simulink model "two_dof_arm_with_lqr"  (R2023a)
settings: Solver=FixedStepAuto  StartTime=0.0  StopTime=5  FixedStep=0.001  RelTol=1e-3
InitFcn:
  | two_link_planar_manipulator_sim
values from neighbouring files (symbols this model uses):
  g = [0 -9.81 0]    [two_link_planar_manipulator_sim.m]
  K = lqr(A,B,Q,R)    [two_link_planar_manipulator_sim.m]
  l = [0.25 0.25]    [two_link_planar_manipulator_sim.m]
  m = [1 1]    [two_link_planar_manipulator_sim.m]
  offset_error = 0.0175    [two_link_planar_manipulator_sim.m]
  resolution = 2^12    (= 4096)    [two_link_planar_manipulator_sim.m]
  sample_time = 0.001    [two_link_planar_manipulator_sim.m]
  true_delay = floor(delay*10^-3/sample_time)+sample_time*10^3    [two_link_planar_manipulator_sim.m]
  w = [0.04 0.04]    [two_link_planar_manipulator_sim.m]
  without_actuator_dynamics = true    [two_link_planar_manipulator_sim.m]
  without_meas_uncertainty = false    [two_link_planar_manipulator_sim.m]
libraries: spsFirstOrderFilterLib x2, robotmaniplib x1, simulink x1
settings Model: Creator=Jordan  LastModifiedBy=Jordan

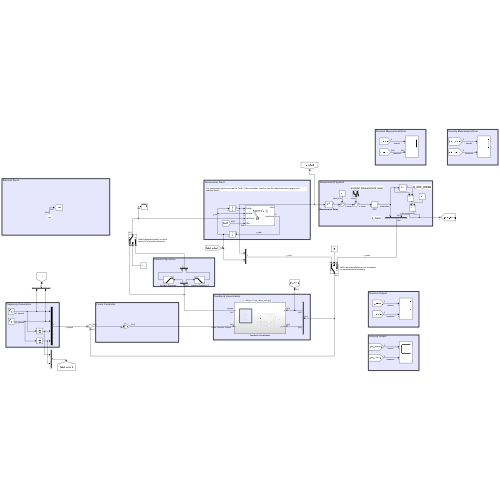
[thumbnail: Simulink's stored preview of the top-level diagram]
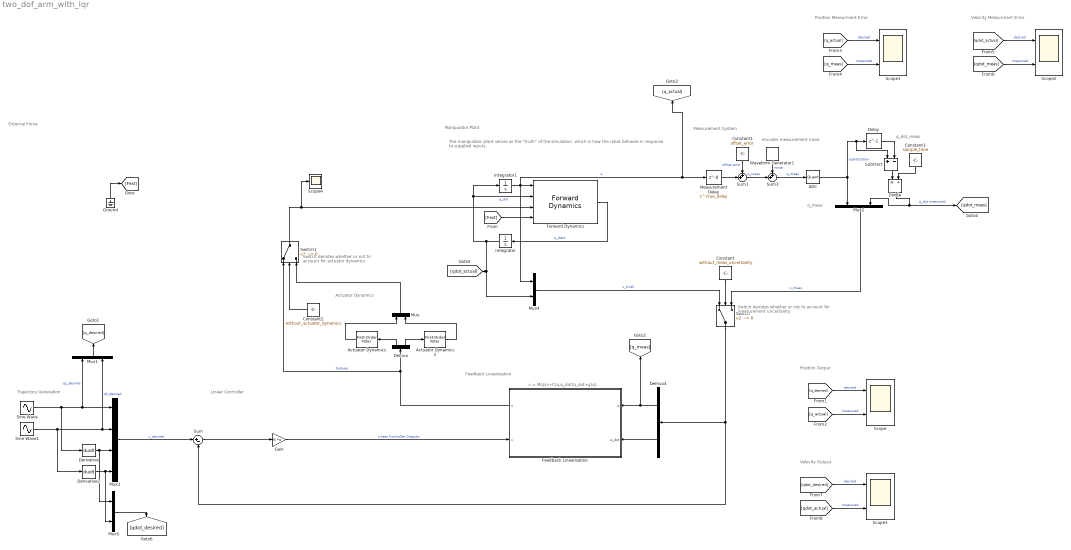
== system two_dof_arm_with_lqr ==
  note: Position Output
  note: Actuator Dynamics
  note: Switch denotes whether or not to account for actuator dynamics
  note: Switch denotes whether or not to account for measurement uncertainty
  note: u = M(q)v+C(q,q_dot)q_dot+g(q)
  note: Manipulator Plant
  note: The manipulator plant serves as the "truth" of the simulation, which is how the robot behaves in response to supplied inputs.
  note: Trajectory Generation
  note: Linear Controller
  note: Measurement System
  note: q_dot_meas
  note: encoder measurement noise
  note: q_meas
  note: Feedback Linearization
  note: External Force
  note: Position Measurment Error
  note: Velocity Measurment Error
  note: Velocity Output
  ADC : Quantizer  QuantizationInterval=2*pi/resolution  LinearizeAsGain=off
  Actuator Dynamics : spsFirstOrderFilterLib/First-Order Filter  FilterType=Lowpass  Tc=4.389e-4  Ts=0  Initialize=off  Vac_Init=[0, 0, 60]  Vdc_Init=0  PlotResponse=off  FreqRange="[0,  200,  1]"
  Actuator Dynamics 2 : spsFirstOrderFilterLib/First-Order Filter  FilterType=Lowpass  Tc=4.389e-4  Ts=0  Initialize=off  Vac_Init=[0, 0, 60]  Vdc_Init=0  PlotResponse=off  FreqRange="[0,  200,  1]"
  Constant : Constant  Value=without_meas_uncertainty
  Constant1 : Constant  Value=offset_error
  Constant2 : Constant  Value=without_actuator_dynamics
  Constant3 : Constant  Value=sample_time
  Delay : Delay  DelayLength=1
  Demux : Demux  Outputs=2
  Demux4 : Demux  Outputs=2
  Derivative : Derivative
  Derivative2 : Derivative
  Divide : Product  Inputs=*/
  Feedback Linearization : Subsystem
      settings: PortSchema="{\"entries\":[{\"content\":{\"sides\":[{\"content\":{\"connectorIds\":[\"In1\",\"In2\"]},\"type\":\"ConnectorPlacement.EquallySpacedRectSide\",\"uuid\":\"e20634ac-7282-4506-b427-a1989d27ee42\"},{\"content\":{\"connectorIds\":[\"Out1\",\"In3\"],\"side\":\"RIGHT\"},\"type\":\"ConnectorPlacement.EquallySpacedRectSide\",\"uuid\":\"ff8f2b23-ed86-4124-b979-83474755293e\"},{\"content\":{\"side\":\"TOP\"},\"type\":\"ConnectorPlacement.EquallySpacedRectSide\",\"uuid\":\"75dc970f-ba8d-4ce0-9b15-e79bd05d50ba\"}]},\"type\":\"ConnectorPlacement.EquallySpacedConnector\",\"uuid\":\"cd5a2392-675b-4624-9569-e6445bfb2136\"}],\"packageUris\":[\"http://schema.mathworks.com/mf0/Connector/R2020b\"],\"version\":\"1.0\"}"
  Forward Dynamics : robotmaniplib/Forward Dynamics  RigidBodyTree=robot  SimulateUsing=Interpreted execution
  Gain : Gain  Gain=K  Multiplication=Matrix(K*u)
  Ground : Ground
  Integrator : Integrator  InitialCondition=[0;0]
  Integrator1 : Integrator  InitialCondition=[0;0]
  Measurement Delay : Delay  DelayLength=true_delay
  Mux{,1..2,4..5} (5 alike) : Mux  Inputs=2
  Mux3 : Mux
  Scope{,1..3} (4 alike) : Scope  NumInputPorts=2
  Scope4 : Scope
  Sine Wave : Sin  Amplitude=pi/2  Frequency=pi  SampleTime=0
  Sine Wave1 : Sin  Amplitude=pi/2  Frequency=pi  Phase=pi  SampleTime=0
  Subtract : Sum  Inputs=+-
  Sum : Sum  Inputs=|+-
  Sum1 : Sum  Inputs=++|
  Sum3 : Sum  Inputs=++|
  Switch : Switch  Criteria=u2 ~= 0  SaturateOnIntegerOverflow=off  InputSameDT=off
  Switch1 : Switch  Criteria=u2 ~= 0  SaturateOnIntegerOverflow=off  InputSameDT=off
  Waveform Generator1 : simulink/Sources/Waveform Generator  OutMin=[]  OutMax=[]  OutDataTypeStr=double  SelectedSignal=1  Signals=gaussian(mean,variance, seed)#gaussian(mean,variance, seed)  BlockNames=MultiportSwitch_510e73f99105412#MultiportSwitch_1249e3761ae8455  SampleTime=0.1
  wires:
  Integrator/1 -> [qdot_actual], Mux4/2, Integrator1/1, Forward Dynamics/2  "q_dot"
  Forward Dynamics/1 -> Integrator/1  "q_ddot"
  Integrator1/1 -> Forward Dynamics/1, Mux4/1, Measurement Delay/1, [q_actual]  "q"
  Delay/1 -> Subtract/2
  Sum3/1 -> ADC/1  "q_meas"
  Waveform Generator1/1 -> Sum3/1  "noise"
  Feedback Linearization/1(u) -> Demux/1, Switch1/1  "torques"
  Demux4/1 -> Feedback Linearization/1(q), [q_meas]
  Demux4/2 -> Feedback Linearization/2(q_dot)
  Gain/1 -> Feedback Linearization/3(v)  "Linear Controller Outputs"
  Ground/1 -> [Fext]
  [Fext] -> Forward Dynamics/4
  Sum1/1 -> Sum3/2  "q_meas"
  Constant1/1 -> Sum1/1  "offset error"
  Measurement Delay/1 -> Sum1/2
  ADC/1 -> Subtract/1, Delay/1, Mux2/1  "quantization"
  Sine Wave/1 -> Mux3/1, Mux1/1, Derivative/1  "q1_desired"
  Demux/2 -> Actuator Dynamics 2/1
  Demux/1 -> Actuator Dynamics/1
  Actuator Dynamics/1 -> Mux/1
  Actuator Dynamics 2/1 -> Mux/2
  Mux1/1 -> [q_desired]
  Sine Wave1/1 -> Derivative2/1, Mux3/2, Mux1/2  "q2_desired"
  Derivative/1 -> Mux5/1, Mux3/3
  Derivative2/1 -> Mux5/2, Mux3/4
  Mux3/1 -> Sum/1  "x_desired"
  Sum/1 -> Gain/1
  Mux4/1 -> Switch/1  "x_truth"
  Mux2/1 -> Switch/3  "x_meas"
  Constant/1 -> Switch/2
  Switch/1 -> Demux4/1, Sum/2
  Switch1/1 -> Scope4/1, Forward Dynamics/3
  Constant2/1 -> Switch1/2
  [q_desired] -> Scope/1  "desired"
  [q_actual] -> Scope/2  "measured"
  [q_actual] -> Scope1/1  "desired"
  [q_meas] -> Scope1/2  "measured"
  Subtract/1 -> Divide/1
  Constant3/1 -> Divide/2
  Divide/1 -> [qdot_meas], Mux2/2  "q_dot measured"
  [qdot_meas] -> Scope2/2  "measured"
  [qdot_actual] -> Scope2/1  "desired"
  [qdot_actual] -> Scope3/2  "measured"
  [qdot_desired] -> Scope3/1  "desired"
  Mux5/1 -> [qdot_desired]
  Mux/1 -> Switch1/3

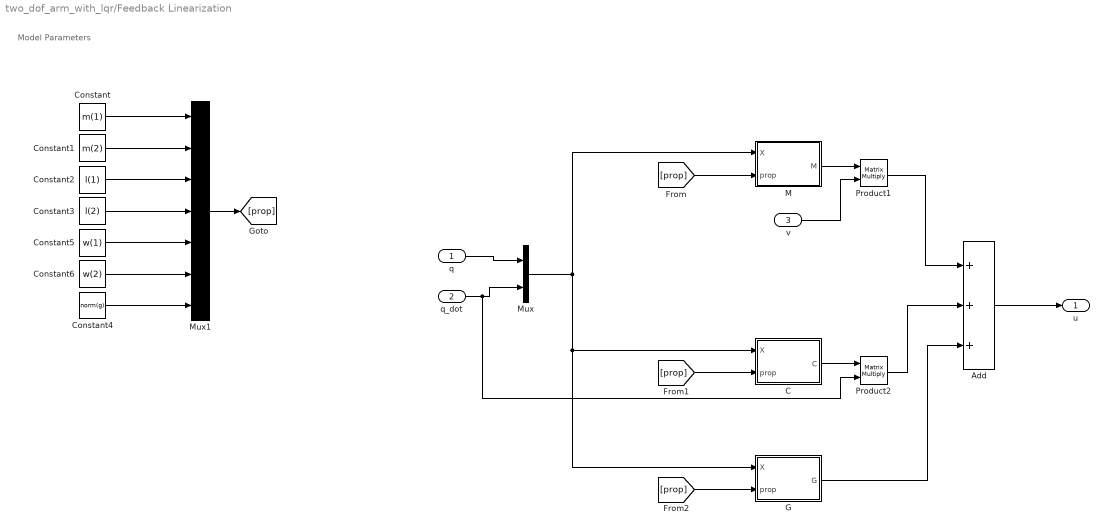
== system two_dof_arm_with_lqr/Feedback Linearization ==
  note: Model Parameters
  q : Inport  PortDimensions=[2 1]
  q_dot : Inport  Port=2  PortDimensions=[2 1]
  v : Inport  Port=3  PortDimensions=[2 1]
  Add : Sum  Inputs=+++
  C : MATLAB Function  TreatAsAtomicUnit=on
  Constant : Constant  Value=m(1)
  Constant1 : Constant  Value=m(2)
  Constant2 : Constant  Value=l(1)
  Constant3 : Constant  Value=l(2)
  Constant4 : Constant  Value=norm(g)
  Constant5 : Constant  Value=w(1)
  Constant6 : Constant  Value=w(2)
  G : MATLAB Function  TreatAsAtomicUnit=on
  M : MATLAB Function  TreatAsAtomicUnit=on
  Mux : Mux  Inputs=2
  Mux1 : Mux  Inputs=7
  Product1 : Product  Multiplication=Matrix(*)
  Product2 : Product  Multiplication=Matrix(*)
  u : Outport  PortDimensions=[2 1]
  wires:
  Constant1/1 -> Mux1/2
  Constant4/1 -> Mux1/7
  Mux1/1 -> [prop]
  Constant/1 -> Mux1/1
  [prop] -> G/2(prop)
  Constant2/1 -> Mux1/3
  [prop] -> C/2(prop)
  Constant3/1 -> Mux1/4
  [prop] -> M/2(prop)
  Mux/1 -> M/1(X), G/1(X), C/1(X)
  q/1 -> Mux/1
  q_dot/1 -> Product2/2, Mux/2
  M/1(M) -> Product1/1
  v/1 -> Product1/2
  Product1/1 -> Add/1
  G/1(G) -> Add/3
  Add/1 -> u/1
  C/1(C) -> Product2/1
  Product2/1 -> Add/2
  Constant5/1 -> Mux1/5
  Constant6/1 -> Mux1/6

== matlab function two_dof_arm_with_lqr/Feedback Linearization/G ==
  data: X input; G output; prop input
function G = fcn(X,prop)
    m1 = prop(1);
    m2 = prop(2);
    l1 = prop(3);
    l2 = prop(4);
    g = prop(7);
    theta1 = X(1);
    theta2 = X(2);
    r1 = l1/2;
    r2 = l2/2;
    
    G1 = g*m2*(r2*cos(theta1+theta2)+l1*cos(theta1))+g*m1*r1*cos(theta1);
    G2 = g*m2*r2*cos(theta1+theta2);
    
    G = [G1;G2];

== matlab function two_dof_arm_with_lqr/Feedback Linearization/M ==
  data: X input; M output; prop input
function M = fcn(X,prop)
    m1 = prop(1);
    m2 = prop(2);
    l1 = prop(3);
    l2 = prop(4);
    w1 = prop(5);
    w2 = prop(6);
    r1 = l1/2;
    r2 = l2/2;
    theta1 = X(1);
    theta2 = X(2);
    Iz1 = 1/12*m1*(l1^2+w1^2);
    Iz2 = 1/12*m2*(l2^2+w2^2);
    
    M11 = m2*l1^2+2*m2*cos(theta2)*l1*r2+m1*r1^2+m2*r2^2+Iz1+Iz2;
    M12 = m2*r2^2+l1*m2*cos(theta2)*r2+Iz2;
    M21 = m2*r2^2+l1*m2*cos(theta2)*r2+Iz2;
    M22 = m2*r2^2+Iz2;
    
    M = [M11 M12; M21 M22];

== matlab function two_dof_arm_with_lqr/Feedback Linearization/C ==
  data: X input; C output; prop input
function C = fcn(X,prop)
    m2 = prop(2);
    l1 = prop(3);
    l2 = prop(4);
    r2 = l2/2;
    theta1 = X(1);
    theta2 = X(2);
    theta1_dot = X(3);
    theta2_dot = X(4);
    
    C11 = -l1*m2*theta2_dot*r2*sin(theta2);
    C12 = -l1*m2*r2*sin(theta2)*(theta1_dot+theta2_dot);
    C21 = l1*m2*theta1_dot*r2*sin(theta2);
    C22 = 0;
    
    C = [C11 C12;C21 C22];
